simulink model "resistors"  (R2024a)
settings: Solver=FixedStepAuto  StartTime=0.0  StopTime=50  FixedStep=1e-3  EnableMultiTasking=on
values from neighbouring files (symbols this model uses):
  wn = 0.5    [PID_controller.m]
  z = 0.3    [PID_controller.m]    (also in P_Controller_RootLocus.m = -log(M/100)/(sqrt(  (pi^2) + (log(M/100))^2  )))
settings Model: ExtModeTrigDuration=2  Creator=DELL  LastModifiedBy=DELL
settings SolverCC: AutoInsertRateTranBlk=on
settings OptimizationCC: EnhancedBackFolding=on  PassReuseOutputArgsAs=Individual arguments  ZeroExternalMemoryAtStartup=off  ZeroInternalMemoryAtStartup=off  MaxStackSize=64  OptimizeBlockOrder=speed  DifferentSizesBufferReuse=on  OptimizationCustomize=off  EfficientTunableParamExpr=on
settings DebuggingCC: ParameterTunabilityLossMsg=error
settings HardwareCC: ProdBitPerInt=16  ProdBitPerPointer=16  ProdBitPerSizeT=16  ProdBitPerPtrDiffT=16  ProdLargestAtomicFloat=None  ProdWordSize=8  ProdHWDeviceType=Atmel->AVR
settings SFSimCC: MATLABDynamicMemAlloc=off
settings RTWCC: Description=Embedded Coder  SystemTargetFile=ert.tlc  HardwareBoard=Arduino Uno  TemplateMakefile=ert_default_tmf  Toolchain=Arduino AVR  BuildConfiguration=Faster Runs
settings CodeAppCC: ForceParamTrailComments=on  IgnoreCustomStorageClasses=off  OperatorAnnotations=on  SimulinkDataObjDesc=on  SFDataObjDesc=on  InsertBlockDesc=on
settings ERTTargetCC: SupportContinuousTime=on  SupportVariableSizeSignals=on  ExtModeTransport=3  ExtModeStaticAlloc=on  ExtModeAutomaticAllocSize=off  ExtModeStaticAllocSize=250  ExtModeMexFile=ext_xcp  ExtModeIntrfLevel=Level2 - Open

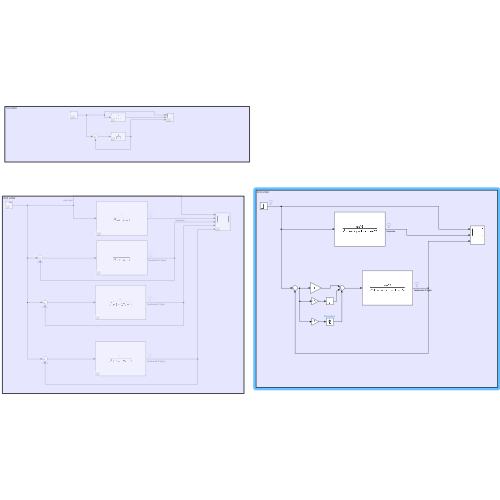
[thumbnail: Simulink's stored preview of the top-level diagram]
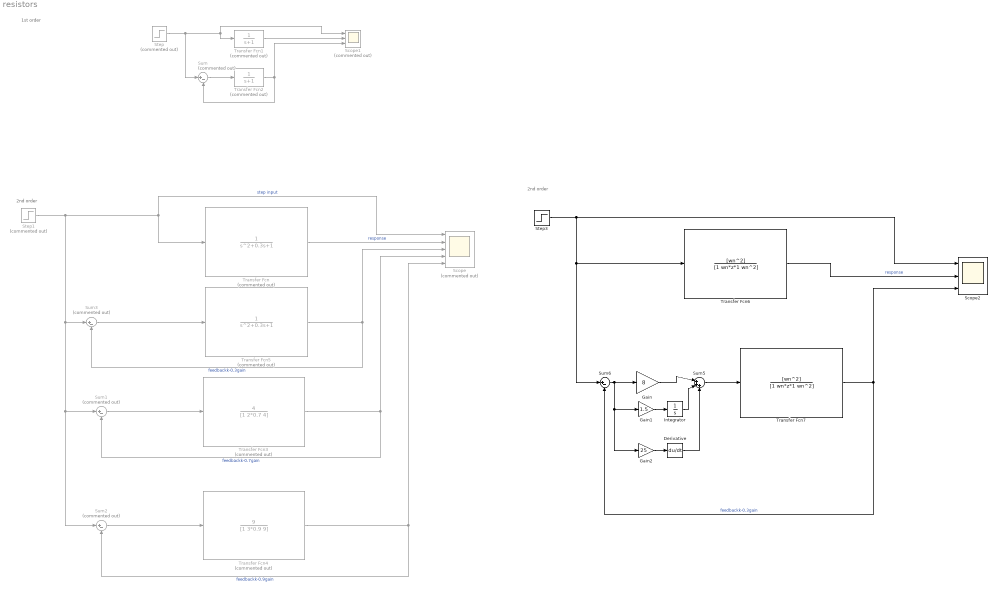
== system resistors ==
  note: 1st order
  note: 2nd order
  note: 2nd order
  Derivative : Derivative
  Gain : Gain  Gain=8
  Gain1 : Gain  Gain=1.5
  Gain2 : Gain  Gain=25
  Integrator : Integrator
  Scope : Scope  Commented=on  NumInputPorts=5
  Scope1 : Scope  Commented=on  NumInputPorts=3
  Scope2 : Scope  NumInputPorts=3
  Step : Step  Commented=on  SampleTime=0
  Step1 : Step  Commented=on  SampleTime=0
  Step3 : Step  SampleTime=0
  Sum{,1..3} (4 alike) : Sum  Commented=on  Inputs=|+-
  Sum5 : Sum  Inputs=|+++
  Sum6 : Sum  Inputs=|+-
  Transfer Fcn : TransferFcn  Commented=on  Numerator=1  Denominator=[1 0.3 1]
  Transfer Fcn1 : TransferFcn  Commented=on  Denominator=[1 1]
  Transfer Fcn2 : TransferFcn  Commented=on  Denominator=[1 1]
  Transfer Fcn3 : TransferFcn  Commented=on  Numerator=4  Denominator=[1 2*0.7 4]
  Transfer Fcn4 : TransferFcn  Commented=on  Numerator=9  Denominator=[1 3*0.9 9]
  Transfer Fcn5 : TransferFcn  Commented=on  Numerator=1  Denominator=[1 0.3 1]
  Transfer Fcn6 : TransferFcn  Numerator=[wn^2]  Denominator=[1 wn*z*1 wn^2]
  Transfer Fcn7 : TransferFcn  Numerator=[wn^2]  Denominator=[1 wn*z*1 wn^2]
  wires:
  Step1/1 -> Scope/1, Transfer Fcn/1, Sum3/1, Sum2/1, Sum1/1  "step input"
  Transfer Fcn/1 -> Scope/2  "response"
  Step/1 -> Sum/1, Scope1/1, Transfer Fcn1/1
  Transfer Fcn2/1 -> Sum/2, Scope1/3
  Transfer Fcn1/1 -> Scope1/2
  Sum/1 -> Transfer Fcn2/1
  Transfer Fcn3/1 -> Scope/4, Sum1/2  "feedbackk-0.7gain"
  Sum1/1 -> Transfer Fcn3/1
  Sum2/1 -> Transfer Fcn4/1
  Transfer Fcn4/1 -> Sum2/2, Scope/5  "feedbackk-0.9gain"
  Transfer Fcn5/1 -> Scope/3, Sum3/2  "feedbackk-0.3gain"
  Sum3/1 -> Transfer Fcn5/1
  Sum6/1 -> Gain2/1, Gain1/1, Gain/1
  Transfer Fcn7/1 -> Sum6/2, Scope2/3  "feedbackk-0.3gain"
  Step3/1 -> Transfer Fcn6/1, Sum6/1, Scope2/1
  Transfer Fcn6/1 -> Scope2/2  "response"
  Gain1/1 -> Integrator/1
  Gain/1 -> Sum5/1
  Integrator/1 -> Sum5/2
  Sum5/1 -> Transfer Fcn7/1
  Gain2/1 -> Derivative/1
  Derivative/1 -> Sum5/3
